simulink model "All_injectors_LQG_plasma_ss_model"  (R2022a)
settings: Solver=FixedStepAuto  StartTime=0.0  StopTime=RunTime  FixedStep=SampleTime  RelTol=1e-3
values from neighbouring files (symbols this model uses):
  K_plasma = dlqr(sys_d_plasma.A, sys_d_plasma.B ,Q_cost_tilde,R_cost, 0)    [All_injectors_LQG_bop_plasma_ss_model_code.m]    (also in All_injectors_LQG_bop_ss_model_code.m = lqr(sys_d_plasma,Q_cost,R_cost); All_injectors_LQG_continuous_time_code.m = lqr(sys_d_plasma,Q_cost,R_cost); All_injectors_LQG_plasma_7_15_24_code.m = lqr(sys_d_plasma,Q_cost,R_cost); All_injectors_LQG_plasma_ss_model_code.m = lqr(sys_d_plasma,Q_cost,R_cost))
  sys_d_plasma = c2d(sysc,dT,'zoh')    [All_injectors_LQG_bop_plasma_ss_model_code.m]    (also in All_injectors_LQG_bop_ss_model_code.m; All_injectors_LQG_continuous_time_code.m; All_injectors_LQG_plasma_7_15_24_code.m; All_injectors_LQG_plasma_ss_model_code.m)
  syskf_plasma = ss(Ad-L*Cd, [Bd L], eye(r), 0*[Bd L], dT)    [All_injectors_LQG_bop_plasma_ss_model_code.m]    (also in All_injectors_LQG_bop_ss_model_code.m = ss(Ad-L*Cd, [Bd L], eye(size_A), 0*[Bd L], dT); All_injectors_LQG_continuous_time_code.m = ss(Ad-L*Cd, [Bd L], eye(size_A), 0*[Bd L], dT); All_injectors_LQG_plasma_7_15_24_code.m = ss(Ad-L*Cd, [Bd L], eye(size_A), 0*[Bd L], dT); All_injectors_LQG_plasma_ss_model_code.m = ss(Ad-L*Cd, [Bd L], eye(size_A), 0*[Bd L], dT))
settings Model: Creator=ducks  LastModifiedBy=ducks
settings DataIOCC: ExternalInput=[t,V]

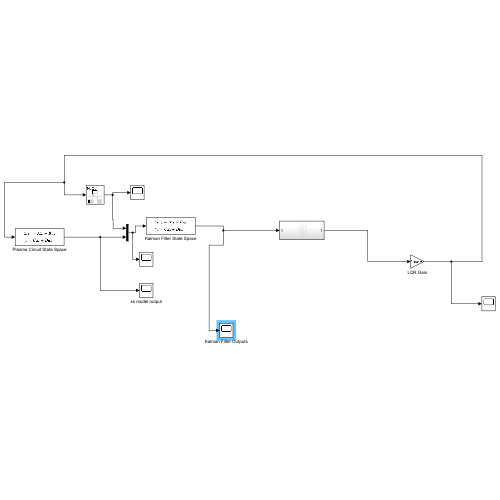
[thumbnail: Simulink's stored preview of the top-level diagram]
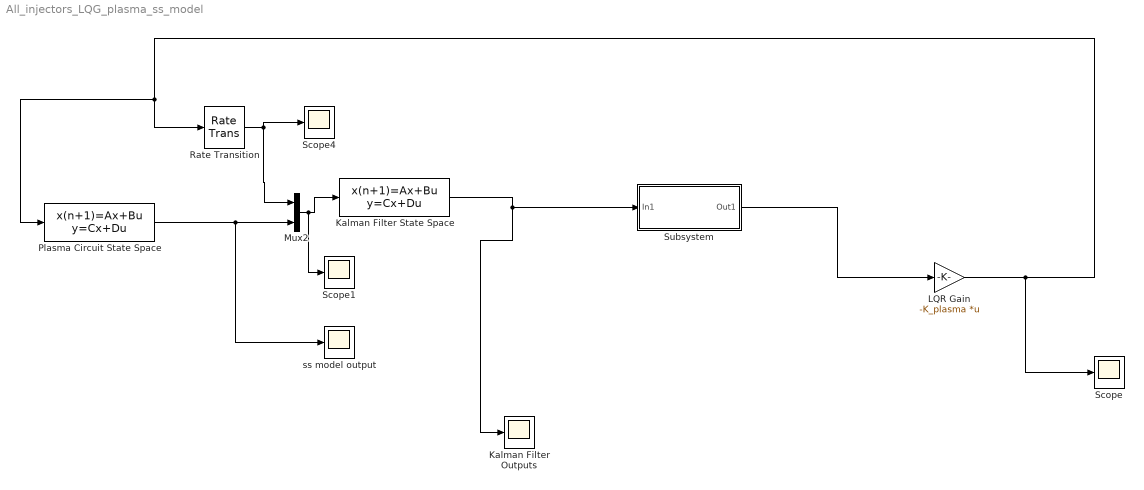
== system All_injectors_LQG_plasma_ss_model ==
  Kalman Filter Outputs : Scope
  Kalman Filter State Space : DiscreteStateSpace  A=syskf_plasma.A  B=syskf_plasma.B  C=syskf_plasma.C  D=syskf_plasma.D  SampleTime=-1
  LQR Gain : Gain  Gain=-K_plasma  Multiplication=Matrix(K*u) (u vector)
  Mux2 : Mux  Inputs=2
  Plasma Circuit State Space : DiscreteStateSpace  A=sys_d_plasma.A  B=sys_d_plasma.B  C=sys_d_plasma.C  D=sys_d_plasma.D  SampleTime=-1
  Rate Transition : RateTransition  OutPortSampleTimeOpt=Inherit
  Scope : Scope
  Scope1 : Scope
  Scope4 : Scope
  Subsystem : Subsystem
  ss model output : Scope
  wires:
  Kalman Filter State Space/1 -> Kalman Filter Outputs/1, Subsystem/1(In1)
  Rate Transition/1 -> Mux2/1, Scope4/1
  Mux2/1 -> Scope1/1, Kalman Filter State Space/1
  Subsystem/1(Out1) -> LQR Gain/1
  LQR Gain/1 -> Scope/1, Rate Transition/1, Plasma Circuit State Space/1
  Plasma Circuit State Space/1 -> ss model output/1, Mux2/2

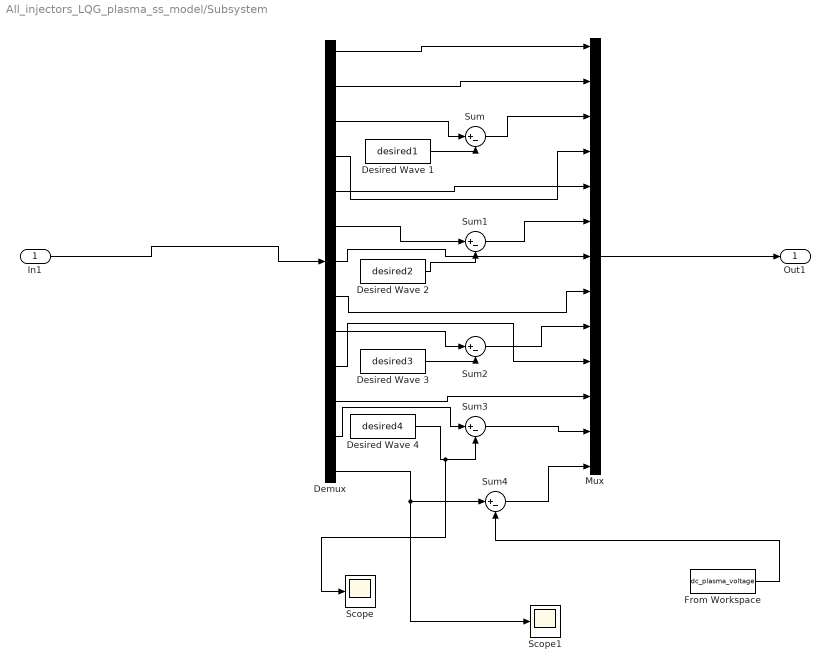
== system All_injectors_LQG_plasma_ss_model/Subsystem ==
  In1 : Inport
  Demux : Demux  Outputs=13
  Desired Wave 1 : FromWorkspace  VariableName=desired1
  Desired Wave 2 : FromWorkspace  VariableName=desired2
  Desired Wave 3 : FromWorkspace  VariableName=desired3
  Desired Wave 4 : FromWorkspace  VariableName=desired4
  From Workspace : FromWorkspace  VariableName=dc_plasma_voltage
  Mux : Mux  Inputs=13
  Scope : Scope
  Scope1 : Scope
  Sum{,1..4} (5 alike) : Sum  Inputs=|+-
  Out1 : Outport
  wires:
  Desired Wave 1/1 -> Sum/2
  Sum1/1 -> Mux/6
  Demux/2 -> Mux/2
  Desired Wave 4/1 -> Scope/1, Sum3/2
  Demux/7 -> Mux/7
  Sum/1 -> Mux/3
  Demux/4 -> Mux/4
  Demux/10 -> Mux/10
  Demux/3 -> Sum/1
  Demux/6 -> Sum1/1
  Demux/8 -> Mux/8
  Demux/1 -> Mux/1
  Sum3/1 -> Mux/12
  Demux/12 -> Sum3/1
  Mux/1 -> Out1/1
  Demux/9 -> Sum2/1
  Demux/5 -> Mux/5
  Desired Wave 2/1 -> Sum1/2
  In1/1 -> Demux/1
  Demux/11 -> Mux/11
  Sum2/1 -> Mux/9
  Desired Wave 3/1 -> Sum2/2
  Demux/13 -> Scope1/1, Sum4/1
  Sum4/1 -> Mux/13
  From Workspace/1 -> Sum4/2
